simulink model "Roboti"  (Simulink 7.9)
settings: Solver=ode45  StartTime=0.0  StopTime=n  RelTol=1e-3
libraries: cstblocks x6
settings Model: Creator=Saeed  LastModifiedBy=Saeed

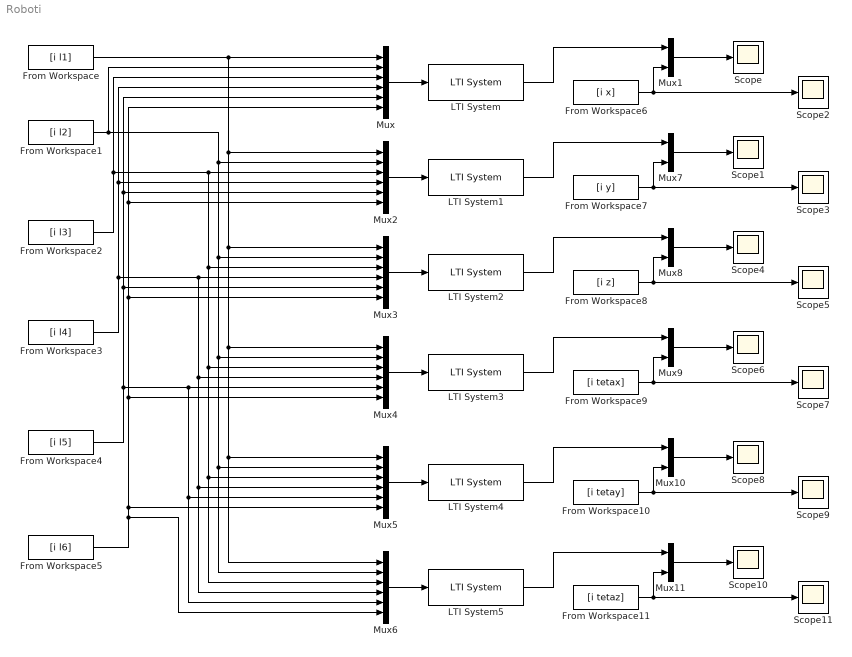
== system Roboti ==
  From Workspace : FromWorkspace  VariableName=[i l1]  SampleTime=0.1
  From Workspace1 : FromWorkspace  VariableName=[i l2]  SampleTime=0.1
  From Workspace10 : FromWorkspace  VariableName=[i tetay]  SampleTime=0.1
  From Workspace11 : FromWorkspace  VariableName=[i tetaz]  SampleTime=0.1
  From Workspace2 : FromWorkspace  VariableName=[i l3]  SampleTime=0.1
  From Workspace3 : FromWorkspace  VariableName=[i l4]  SampleTime=0.1
  From Workspace4 : FromWorkspace  VariableName=[i l5]  SampleTime=0.1
  From Workspace5 : FromWorkspace  VariableName=[i l6]  SampleTime=0.1
  From Workspace6 : FromWorkspace  VariableName=[i x]  SampleTime=0.1
  From Workspace7 : FromWorkspace  VariableName=[i y]  SampleTime=0.1
  From Workspace8 : FromWorkspace  VariableName=[i z]  SampleTime=0.1
  From Workspace9 : FromWorkspace  VariableName=[i tetax]  SampleTime=0.1
  LTI System : cstblocks/LTI System  sys=Xss5  IC=0.077441335304176
  LTI System1 : cstblocks/LTI System  sys=Yss5  IC=[]
  LTI System2 : cstblocks/LTI System  sys=Zss5  IC=[]
  LTI System3 : cstblocks/LTI System  sys=tXss5  IC=[]
  LTI System4 : cstblocks/LTI System  sys=tYss5  IC=[]
  LTI System5 : cstblocks/LTI System  sys=tZss5  IC=[]
  Mux{,2..6} (6 alike) : Mux  Inputs=6
  Mux{1,7..11} (6 alike) : Mux  Inputs=2
  Scope{,1..11} (12 alike) : Scope
      Scope10 settings: SaveName=ScopeData10
      Scope11 settings: SaveName=ScopeData11
      Scope2 settings: SaveName=ScopeData2
      Scope3 settings: SaveName=ScopeData3
      Scope4 settings: SaveName=ScopeData4
      Scope5 settings: SaveName=ScopeData5
      Scope6 settings: TimeRange=12000  YMin=-0.1  YMax=0.6000000000000001  SaveName=ScopeData6
      Scope7 settings: SaveName=ScopeData7
      Scope8 settings: SaveName=ScopeData8
      Scope9 settings: SaveName=ScopeData9
  wires:
  Mux/1 -> LTI System/1
  Mux1/1 -> Scope/1
  From Workspace6/1 -> Mux1/2, Scope2/1
  Mux2/1 -> LTI System1/1
  Mux3/1 -> LTI System2/1
  Mux4/1 -> LTI System3/1
  Mux5/1 -> LTI System4/1
  Mux6/1 -> LTI System5/1
  From Workspace/1 -> Mux/1, Mux2/1, Mux3/1, Mux4/1, Mux5/1, Mux6/1
  From Workspace1/1 -> Mux/2, Mux2/2, Mux3/2, Mux4/2, Mux5/2, Mux6/2
  From Workspace5/1 -> Mux/6, Mux2/6, Mux3/6, Mux4/6, Mux5/6, Mux6/6
  Mux7/1 -> Scope1/1
  From Workspace7/1 -> Mux7/2, Scope3/1
  Mux8/1 -> Scope4/1
  From Workspace8/1 -> Mux8/2, Scope5/1
  Mux9/1 -> Scope6/1
  From Workspace9/1 -> Mux9/2, Scope7/1
  Mux10/1 -> Scope8/1
  From Workspace10/1 -> Mux10/2, Scope9/1
  Mux11/1 -> Scope10/1
  From Workspace11/1 -> Mux11/2, Scope11/1
  LTI System/1 -> Mux1/1
  LTI System1/1 -> Mux7/1
  LTI System2/1 -> Mux8/1
  LTI System3/1 -> Mux9/1
  LTI System4/1 -> Mux10/1
  LTI System5/1 -> Mux11/1
  From Workspace2/1 -> Mux/3, Mux2/3, Mux3/3, Mux4/3, Mux5/3, Mux6/3
  From Workspace3/1 -> Mux/4, Mux2/4, Mux3/4, Mux4/4, Mux5/4, Mux6/4
  From Workspace4/1 -> Mux/5, Mux2/5, Mux3/5, Mux4/5, Mux5/5, Mux6/5
